simulink model "part1_1"  (R2023b)
settings: Solver=VariableStepAuto  StartTime=0.0  StopTime=10.0  RelTol=1e-3
settings Model: Creator=Zahedi  LastModifiedBy=Zahedi

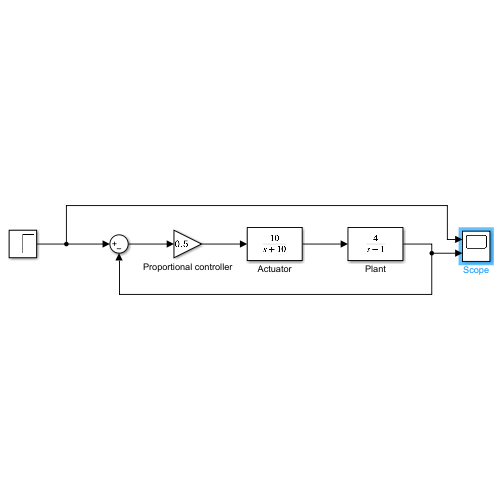
[thumbnail: Simulink's stored preview of the top-level diagram]
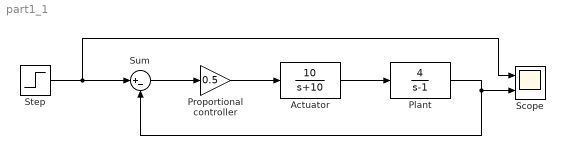
== system part1_1 ==
  Actuator : TransferFcn  Numerator=[10]  Denominator=[1 10]
  Plant : TransferFcn  Numerator=[4]  Denominator=[1 -1]
  Proportional controller : Gain  Gain=0.5
  Scope : Scope  NumInputPorts=2
  Step : Step  SampleTime=0
  Sum : Sum  Inputs=|+-
  wires:
  Actuator/1 -> Plant/1
  Proportional controller/1 -> Actuator/1
  Plant/1 -> Sum/2, Scope/2
  Sum/1 -> Proportional controller/1
  Step/1 -> Scope/1, Sum/1
